simulink model "RS232ex6"  (Simulink 5.0)
settings: Solver=ode1  StartTime=0.0  StopTime=10.0  FixedStep=1  RelTol=1e-3
undefined symbols (not defined in the file or in its folder): _00594
libraries: RS232 x3
settings Model: LastModifiedBy=leo

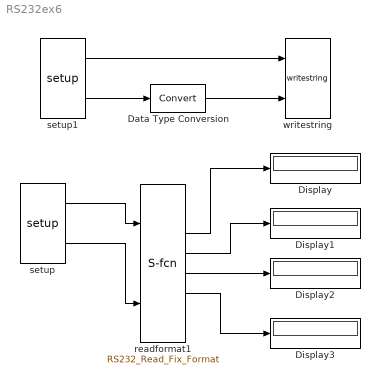
== system RS232ex6 ==
  Data Type Conversion : DataTypeConversion  SaturateOnIntegerOverflow=on
  Display{,1..3} (4 alike) : Display
  readformat1 : S-Function  AncestorBlock=RS232/readformat1  FunctionName=RS232_Read_Fix_Format  Parameters=fmtString,sampTime  mask(readformat){fmtString=_%5i4%%4i4%%4i4%%3i4%%3i4%%3i4%_, sampTime=-1}
      mask prompts: fmtString "Format String"; sampTime "Sample time"
      mask help: RS232 Read Format
      mask Help: RS232 Read Format
      mask Display: disp('RS232\nRead\nFix\nFormat');
  setup : RS232/setup  port=COM2  baudrate=115200  databit=8  stopbit=1  parity=None
  setup1 : RS232/setup  port=COM1  baudrate=115200  databit=8  stopbit=1  parity=None
  writestring : RS232/writestring  string=_00594-003+000357000000_
  wires:
  readformat1/5 -> Display2/1
  readformat1/4 -> Display1/1
  readformat1/3 -> Display/1
  setup/1 -> readformat1/1
  setup/2 -> readformat1/2
  setup1/2 -> Data Type Conversion/1
  setup1/1 -> writestring/1
  Data Type Conversion/1 -> writestring/2
  readformat1/6 -> Display3/1
